simulink model "VB_RIFKF_GNSS_INS25"  (R2023a)
settings: Solver=FixedStepAuto  StartTime=0  StopTime=500  FixedStep=0.01  RelTol=1e-3
InitFcn:
  | resilient_initNavigation1216;
  | init_param;
undefined symbols (not defined in the file or in its folder): dt, g0, gam0_rad, ISUS_flag, magnitude, p, P0, P0_RIEKF, param, pd0, pe0, phi0_rad, pn0, psi, psi0_rad, state_dim, vd0, ve0, vn0
libraries: simulink_extras x68, dspstat3 x54, sharedtransform x47, simulink x43, matrix_library x9, sharedTrackingLibrary x5, dspfactors x4, aerolibconvert2 x3, aerolibtransform2 x3
(part 16 of 22)

== system VB_RIFKF_GNSS_INS25/ISUS_RIEKF3/INS propogation3/vel//pos update/Kinematic Equation ==
  Cbn : Inport
  Ab : Inport  Port=2
  Add : Sum  Inputs=+-
  Add1 : Sum  Inputs=+-
  Constant : Constant  Value=[0 0 -g0]  OutDataTypeStr=single
  Constant1 : Constant  Value=[0 0 -g0]  OutDataTypeStr=single
  Product : Product  Multiplication=Matrix(*)  RndMeth=Zero
  Product1 : Product  Multiplication=Matrix(*)  RndMeth=Zero
  Scope : Scope
  Scope1 : Scope  NumInputPorts=2
  Transpose : Math  Operator=transpose
  An : Outport
  ab_nog : Outport  Port=2
  wires:
  Cbn/1 -> Transpose/1, Product/1
  Add/1 -> An/1, Scope1/2
  Ab/1 -> Product/2, Add1/1, Scope1/1
  Product/1 -> Scope/1, Add/1
  Constant/1 -> Add/2
  Transpose/1 -> Product1/1  "Cnb"
  Constant1/1 -> Product1/2  "gn"
  Product1/1 -> Add1/2  "gb"
  Add1/1 -> ab_nog/1  "ab_nog"

== system VB_RIFKF_GNSS_INS25/ISUS_RIEKF3/INS propogation3/vel//pos update/pos update ==
  dtheta : Inport
  vel_k : Inport  Port=2
  dp : Inport  Port=3
  QGC_init : Inport  Port=4
  p0 : Inport  Port=5
  Add1 : Sum
  Delay1 : Delay  DelayLength=1  InitialConditionSource=Input port  ExternalReset=Rising
      settings: InputPortMap=u0,r5,p4
  Gain1 : Gain  Gain=dt
  MATLAB Function : MATLAB Function  TreatAsAtomicUnit=on
  Reshape1 : Reshape  OutputDimensionality=Column vector (2-D)
  p_k : Outport
  wires:
  p0/1 -> Reshape1/1
  QGC_init/1 -> Delay1/2
  Reshape1/1 -> Delay1/3
  Delay1/1 -> Add1/2
  Gain1/1 -> Add1/1
  vel_k/1 -> Gain1/1
  dtheta/1 -> MATLAB Function/1(dtheta)
  dp/1 -> MATLAB Function/2(KFState_dp)
  Add1/1 -> MATLAB Function/3(pos)
  MATLAB Function/1(pos_correct) -> Delay1/1, p_k/1

== system VB_RIFKF_GNSS_INS25/ISUS_RIEKF3/INS propogation3/vel//pos update/vel update ==
  dtheta : Inport
  QGC_init : Inport  Port=2
  An : Inport  Port=3
  KFState_dv : Inport  Port=4
  v0 : Inport  Port=5
  Add : Sum
  Delay : Delay  DelayLength=1  InitialConditionSource=Input port  ExternalReset=Rising
      settings: InputPortMap=u0,r5,p4
  Gain : Gain  Gain=dt
  MATLAB Function : MATLAB Function  TreatAsAtomicUnit=on
  Reshape : Reshape  OutputDimensionality=Column vector (2-D)
  vel_k : Outport
  wires:
  QGC_init/1 -> Delay/2
  Reshape/1 -> Delay/3
  An/1 -> Gain/1
  v0/1 -> Reshape/1
  Gain/1 -> Add/1
  Delay/1 -> Add/2
  KFState_dv/1 -> MATLAB Function/2(KFState_dv)
  dtheta/1 -> MATLAB Function/1(dtheta)
  Add/1 -> MATLAB Function/3(vel)
  MATLAB Function/1(vel_correct) -> Delay/1, vel_k/1

== system VB_RIFKF_GNSS_INS25/No.1_Sensor_Data_Process/IMU_Data_Process/Bias Eliminate/Subsystem ==
  data : Inport
  Buffer : Buffer  N=50  V=49  OutputFrames=off
  Buffer1 : Buffer  N=50  V=49  OutputFrames=off
  Buffer2 : Buffer  N=50  V=49  OutputFrames=off
  Demux : Demux  Outputs=3
  Mean4 : dspstat3/Mean  run=off  reset_popup=None  directionMode=Entire input  dimension=3  roiEnable=off  roiType=Rectangles  roiPortion=Entire ROI  roiOutput=Individual statistics for each ROI  roiFlag=off  roundingMode=Floor  overflowMode=off  outputDataTypeStr=Inherit: Same as accumulator  outputMin=[]  outputMax=[]  outputLastDataTypeStr=Inherit: Same as accumulator
  Mean5 : dspstat3/Mean  run=off  reset_popup=None  directionMode=Entire input  dimension=3  roiEnable=off  roiType=Rectangles  roiPortion=Entire ROI  roiOutput=Individual statistics for each ROI  roiFlag=off  roundingMode=Floor  overflowMode=off  outputDataTypeStr=Inherit: Same as accumulator  outputMin=[]  outputMax=[]  outputLastDataTypeStr=Inherit: Same as accumulator
  Mean6 : dspstat3/Mean  run=off  reset_popup=None  directionMode=Entire input  dimension=3  roiEnable=off  roiType=Rectangles  roiPortion=Entire ROI  roiOutput=Individual statistics for each ROI  roiFlag=off  roundingMode=Floor  overflowMode=off  outputDataTypeStr=Inherit: Same as accumulator  outputMin=[]  outputMax=[]  outputLastDataTypeStr=Inherit: Same as accumulator
  Scope : Scope  NumInputPorts=2
  Vector Concatenate : Concatenate  NumInputs=3
  mean_data : Outport
  wires:
  data/1 -> Demux/1, Scope/1
  Vector Concatenate/1 -> mean_data/1, Scope/2
  Mean4/1 -> Vector Concatenate/1
  Demux/3 -> Buffer2/1
  Buffer1/1 -> Mean5/1  "fby_buff"
  Demux/1 -> Buffer/1
  Buffer2/1 -> Mean6/1  "fbz_buff"
  Mean5/1 -> Vector Concatenate/2
  Buffer/1 -> Mean4/1  "fbx_buff"
  Demux/2 -> Buffer1/1
  Mean6/1 -> Vector Concatenate/3

== system VB_RIFKF_GNSS_INS25/No.1_Sensor_Data_Process1/IMU_Data_Process/Bias Eliminate/Subsystem ==
  data : Inport
  Buffer : Buffer  N=50  V=49  OutputFrames=off
  Buffer1 : Buffer  N=50  V=49  OutputFrames=off
  Buffer2 : Buffer  N=50  V=49  OutputFrames=off
  Demux : Demux  Outputs=3
  Mean4 : dspstat3/Mean  run=off  reset_popup=None  directionMode=Entire input  dimension=3  roiEnable=off  roiType=Rectangles  roiPortion=Entire ROI  roiOutput=Individual statistics for each ROI  roiFlag=off  roundingMode=Floor  overflowMode=off  outputDataTypeStr=Inherit: Same as accumulator  outputMin=[]  outputMax=[]  outputLastDataTypeStr=Inherit: Same as accumulator
  Mean5 : dspstat3/Mean  run=off  reset_popup=None  directionMode=Entire input  dimension=3  roiEnable=off  roiType=Rectangles  roiPortion=Entire ROI  roiOutput=Individual statistics for each ROI  roiFlag=off  roundingMode=Floor  overflowMode=off  outputDataTypeStr=Inherit: Same as accumulator  outputMin=[]  outputMax=[]  outputLastDataTypeStr=Inherit: Same as accumulator
  Mean6 : dspstat3/Mean  run=off  reset_popup=None  directionMode=Entire input  dimension=3  roiEnable=off  roiType=Rectangles  roiPortion=Entire ROI  roiOutput=Individual statistics for each ROI  roiFlag=off  roundingMode=Floor  overflowMode=off  outputDataTypeStr=Inherit: Same as accumulator  outputMin=[]  outputMax=[]  outputLastDataTypeStr=Inherit: Same as accumulator
  Scope : Scope  NumInputPorts=2
  Vector Concatenate : Concatenate  NumInputs=3
  mean_data : Outport
  wires:
  Mean6/1 -> Vector Concatenate/3
  Demux/2 -> Buffer1/1
  Buffer/1 -> Mean4/1  "fbx_buff"
  Mean5/1 -> Vector Concatenate/2
  Buffer2/1 -> Mean6/1  "fbz_buff"
  Demux/1 -> Buffer/1
  Buffer1/1 -> Mean5/1  "fby_buff"
  Demux/3 -> Buffer2/1
  Mean4/1 -> Vector Concatenate/1
  Vector Concatenate/1 -> Scope/2, mean_data/1
  data/1 -> Scope/1, Demux/1

== system VB_RIFKF_GNSS_INS25/No.1_Sensor_Data_Process2/IMU_Data_Process/Bias Eliminate/Subsystem ==
  data : Inport
  Buffer : Buffer  N=50  V=49  OutputFrames=off
  Buffer1 : Buffer  N=50  V=49  OutputFrames=off
  Buffer2 : Buffer  N=50  V=49  OutputFrames=off
  Demux : Demux  Outputs=3
  Mean4 : dspstat3/Mean  run=off  reset_popup=None  directionMode=Entire input  dimension=3  roiEnable=off  roiType=Rectangles  roiPortion=Entire ROI  roiOutput=Individual statistics for each ROI  roiFlag=off  roundingMode=Floor  overflowMode=off  outputDataTypeStr=Inherit: Same as accumulator  outputMin=[]  outputMax=[]  outputLastDataTypeStr=Inherit: Same as accumulator
  Mean5 : dspstat3/Mean  run=off  reset_popup=None  directionMode=Entire input  dimension=3  roiEnable=off  roiType=Rectangles  roiPortion=Entire ROI  roiOutput=Individual statistics for each ROI  roiFlag=off  roundingMode=Floor  overflowMode=off  outputDataTypeStr=Inherit: Same as accumulator  outputMin=[]  outputMax=[]  outputLastDataTypeStr=Inherit: Same as accumulator
  Mean6 : dspstat3/Mean  run=off  reset_popup=None  directionMode=Entire input  dimension=3  roiEnable=off  roiType=Rectangles  roiPortion=Entire ROI  roiOutput=Individual statistics for each ROI  roiFlag=off  roundingMode=Floor  overflowMode=off  outputDataTypeStr=Inherit: Same as accumulator  outputMin=[]  outputMax=[]  outputLastDataTypeStr=Inherit: Same as accumulator
  Scope : Scope  NumInputPorts=2
  Vector Concatenate : Concatenate  NumInputs=3
  mean_data : Outport
  wires:
  data/1 -> Demux/1, Scope/1
  Vector Concatenate/1 -> mean_data/1, Scope/2
  Mean4/1 -> Vector Concatenate/1
  Demux/3 -> Buffer2/1
  Buffer1/1 -> Mean5/1  "fby_buff"
  Demux/1 -> Buffer/1
  Buffer2/1 -> Mean6/1  "fbz_buff"
  Mean5/1 -> Vector Concatenate/2
  Buffer/1 -> Mean4/1  "fbx_buff"
  Demux/2 -> Buffer1/1
  Mean6/1 -> Vector Concatenate/3

== system VB_RIFKF_GNSS_INS25/ER EKF/Error State Kalman Filter/Extended Kalman Filter1/Correct1/Sk_m_innovation ==
  Pk/k_1 : Inport
  yMeas : Inport  Port=2
  X : Inport  Port=3
  R : Inport  Port=4
  Abs : Abs  Commented=on  SaturateOnIntegerOverflow=off
  Abs1 : Abs  SaturateOnIntegerOverflow=off
  Add : Sum
  Add1 : Sum  Inputs=+-
  Add2 : Sum
  Constant : Constant  Commented=on  Value=8
  Constant1 : Constant  Commented=on  Value=8
  Constant2 : Constant  Commented=on  Value=12
  Constant3 : Constant  Value=eps
  Constant4 : Constant  Commented=on  Value=15
  Constant5 : Constant  Commented=on  Value=8
  Constant6 : Constant  Value=[eye(6),zeros(6,9)]  OutDataTypeStr=single
  Constant7 : Constant  Commented=on  Value=15
  Constant8 : Constant  Commented=on  Value=12
  Constant9 : Constant  Commented=on  Value=25
  Divide : Product  Inputs=*/
  Extract Diagonal1 : matrix_library/Extract Diagonal
  MATLAB Function : MATLAB Function  Commented=on  TreatAsAtomicUnit=on
  Product : Product  Inputs=3  Multiplication=Matrix(*)
  Product1 : Product  Multiplication=Matrix(*)
  Product2 : Product  Commented=on
  Scope : Scope
  Sqrt1 : Sqrt
  Transpose : Math  Operator=transpose
  yMeas1 : InportShadow  Port=2
  measurement innovation : Outport
  wires:
  Product/1 -> Add/1
  Transpose/1 -> Product/3
  R/1 -> Add/2
  Pk/k_1/1 -> Product/2
  yMeas/1 -> Add1/1
  Constant6/1 -> Product1/1, Product/1, Transpose/1
  X/1 -> Product1/2
  Product1/1 -> Add1/2
  Add/1 -> Extract Diagonal1/1  "S"
  Divide/1 -> measurement innovation/1, Abs/1, Scope/1
  MATLAB Function/1(w) -> Product2/1
  Extract Diagonal1/1 -> Abs1/1
  Add1/1 -> Divide/1
  Sqrt1/1 -> Add2/1
  Abs/1 -> MATLAB Function/1(err)
  Abs1/1 -> Sqrt1/1
  Add2/1 -> Divide/2
  Constant3/1 -> Add2/2
  yMeas1/1 -> Product2/2
  Constant1/1 -> MATLAB Function/2(k0)
  Constant4/1 -> MATLAB Function/3(k1)
  Constant/1 -> MATLAB Function/4(zk0)
  Constant2/1 -> MATLAB Function/5(zk1)

== system VB_RIFKF_GNSS_INS25/ER EKF/Error State Kalman Filter/Extended Kalman Filter1/Predict/If Action Subsystem ==
  Action Port : ActionPort
  Constant : Constant  Value=0
  Data Store Read : DataStoreRead  DataStoreName=x  IndexOptions=Index vector (dialog)  Indices=1  OutputSizes=1
  Data Store Write : DataStoreWrite  DataStoreName=x  IndexOptions=Index vector (dialog)  Indices=1  OutputSizes=1
  Data Store Write1 : DataStoreWrite  DataStoreName=feedback_flag_18dim  IndexOptions=Index vector (dialog)  Indices=1  OutputSizes=1
  Mux : Mux  Inputs=2
  Selector : Selector  InputPortWidth=18  IndexOptions=Index vector (dialog)  Indices=[16 17 18]  OutputSizes=1
  Zero : Constant  Value=zeros(15,1)  OutDataTypeStr=Inherit: Inherit via back propagation
  wires:
  Constant/1 -> Data Store Write1/1
  Data Store Read/1 -> Selector/1
  Zero/1 -> Mux/1
  Selector/1 -> Mux/2
  Mux/1 -> Data Store Write/1

== system VB_RIFKF_GNSS_INS25/ER EKF/Error State Kalman Filter/Extended Kalman Filter2/Correct1/Sk_m_innovation ==
  Pk/k_1 : Inport
  yMeas : Inport  Port=2
  X : Inport  Port=3
  R : Inport  Port=4
  Abs : Abs  Commented=on  SaturateOnIntegerOverflow=off
  Abs1 : Abs  SaturateOnIntegerOverflow=off
  Add : Sum
  Add1 : Sum  Inputs=+-
  Add2 : Sum
  Constant : Constant  Commented=on  Value=8
  Constant1 : Constant  Commented=on  Value=8
  Constant2 : Constant  Commented=on  Value=12
  Constant3 : Constant  Value=eps
  Constant4 : Constant  Commented=on  Value=15
  Constant5 : Constant  Commented=on  Value=8
  Constant6 : Constant  Value=[eye(6),zeros(6,9)]  OutDataTypeStr=single
  Constant7 : Constant  Commented=on  Value=15
  Constant8 : Constant  Commented=on  Value=12
  Constant9 : Constant  Commented=on  Value=25
  Divide : Product  Inputs=*/
  Extract Diagonal1 : matrix_library/Extract Diagonal
  MATLAB Function : MATLAB Function  Commented=on  TreatAsAtomicUnit=on
  Product : Product  Inputs=3  Multiplication=Matrix(*)
  Product1 : Product  Multiplication=Matrix(*)
  Product2 : Product  Commented=on
  Scope : Scope
  Sqrt1 : Sqrt
  Transpose : Math  Operator=transpose
  yMeas1 : InportShadow  Port=2
  measurement innovation : Outport
  wires:
  Product/1 -> Add/1
  Transpose/1 -> Product/3
  R/1 -> Add/2
  Pk/k_1/1 -> Product/2
  yMeas/1 -> Add1/1
  Constant6/1 -> Product1/1, Product/1, Transpose/1
  X/1 -> Product1/2
  Product1/1 -> Add1/2
  Add/1 -> Extract Diagonal1/1  "S"
  Divide/1 -> measurement innovation/1, Abs/1, Scope/1
  MATLAB Function/1(w) -> Product2/1
  Extract Diagonal1/1 -> Abs1/1
  Add1/1 -> Divide/1
  Sqrt1/1 -> Add2/1
  Abs/1 -> MATLAB Function/1(err)
  Abs1/1 -> Sqrt1/1
  Add2/1 -> Divide/2
  Constant3/1 -> Add2/2
  yMeas1/1 -> Product2/2
  Constant1/1 -> MATLAB Function/2(k0)
  Constant4/1 -> MATLAB Function/3(k1)
  Constant/1 -> MATLAB Function/4(zk0)
  Constant2/1 -> MATLAB Function/5(zk1)

== system VB_RIFKF_GNSS_INS25/ER EKF/Error State Kalman Filter/Extended Kalman Filter2/Predict/If Action Subsystem ==
  Action Port : ActionPort
  Constant : Constant  Value=0
  Data Store Read : DataStoreRead  DataStoreName=x  IndexOptions=Index vector (dialog)  Indices=1  OutputSizes=1
  Data Store Write : DataStoreWrite  DataStoreName=x  IndexOptions=Index vector (dialog)  Indices=1  OutputSizes=1
  Data Store Write1 : DataStoreWrite  DataStoreName=feedback_flag_18dim  IndexOptions=Index vector (dialog)  Indices=1  OutputSizes=1
  Mux : Mux  Inputs=2
  Selector : Selector  InputPortWidth=18  IndexOptions=Index vector (dialog)  Indices=[16 17 18]  OutputSizes=1
  Zero : Constant  Value=zeros(15,1)  OutDataTypeStr=Inherit: Inherit via back propagation
  wires:
  Constant/1 -> Data Store Write1/1
  Data Store Read/1 -> Selector/1
  Zero/1 -> Mux/1
  Selector/1 -> Mux/2
  Mux/1 -> Data Store Write/1

== system VB_RIFKF_GNSS_INS25/ER EKF/INS propogation/Init_PVQ/Horizontal_attitude/Deal with zero ==
  In1 : Inport
  Add5 : Sum
  Constant1 : Constant  Value=1e-6  OutDataTypeStr=single
  Out1 : Outport
  wires:
  Constant1/1 -> Add5/2
  In1/1 -> Add5/1
  Add5/1 -> Out1/1

== system VB_RIFKF_GNSS_INS25/ER EKF/INS propogation/Init_PVQ/Horizontal_attitude2/Deal with zero ==
  In1 : Inport
  Add5 : Sum
  Constant1 : Constant  Value=1e-6  OutDataTypeStr=single
  Out1 : Outport
  wires:
  Constant1/1 -> Add5/2
  In1/1 -> Add5/1
  Add5/1 -> Out1/1

== system VB_RIFKF_GNSS_INS25/ER EKF/INS propogation/gyro bias compensation/error compensation/If Action Subsystem1 ==
  Action Port : ActionPort  ActionPortLabel=if(u1 == 1)
  Constant : Constant
  Data Store Write : DataStoreWrite  DataStoreName=feedback_flag_18dim  IndexOptions=Index vector (dialog)  Indices=1  OutputSizes=1
  wires:
  Constant/1 -> Data Store Write/1

== system VB_RIFKF_GNSS_INS25/ISUS_RIEKF1/Error State Kalman Filter M1/Extended Kalman Filter M1/Predict/If Action Subsystem ==
  Action Port : ActionPort
  Constant : Constant  Value=0
  Data Store Read : DataStoreRead  DataStoreName=x  IndexOptions=Index vector (dialog)  Indices=1  OutputSizes=1
  Data Store Write : DataStoreWrite  DataStoreName=x  IndexOptions=Index vector (dialog)  Indices=1  OutputSizes=1
  Data Store Write1 : DataStoreWrite  DataStoreName=feedback_flag_18dim  IndexOptions=Index vector (dialog)  Indices=1  OutputSizes=1
  Mux : Mux  Inputs=2
  Selector : Selector  InputPortWidth=18  IndexOptions=Index vector (dialog)  Indices=[16 17 18]  OutputSizes=1
  Zero : Constant  Value=zeros(15,1)  OutDataTypeStr=Inherit: Inherit via back propagation
  wires:
  Constant/1 -> Data Store Write1/1
  Data Store Read/1 -> Selector/1
  Zero/1 -> Mux/1
  Selector/1 -> Mux/2
  Mux/1 -> Data Store Write/1

== system VB_RIFKF_GNSS_INS25/ISUS_RIEKF1/Error State Kalman Filter M1/Extended Kalman Filter M2/Predict/If Action Subsystem ==
  Action Port : ActionPort
  Constant : Constant  Value=0
  Data Store Read : DataStoreRead  DataStoreName=x  IndexOptions=Index vector (dialog)  Indices=1  OutputSizes=1
  Data Store Write : DataStoreWrite  DataStoreName=x  IndexOptions=Index vector (dialog)  Indices=1  OutputSizes=1
  Data Store Write1 : DataStoreWrite  DataStoreName=feedback_flag_18dim  IndexOptions=Index vector (dialog)  Indices=1  OutputSizes=1
  Mux : Mux  Inputs=2
  Selector : Selector  InputPortWidth=18  IndexOptions=Index vector (dialog)  Indices=[16 17 18]  OutputSizes=1
  Zero : Constant  Value=zeros(15,1)  OutDataTypeStr=Inherit: Inherit via back propagation
  wires:
  Mux/1 -> Data Store Write/1
  Selector/1 -> Mux/2
  Zero/1 -> Mux/1
  Data Store Read/1 -> Selector/1
  Constant/1 -> Data Store Write1/1

== system VB_RIFKF_GNSS_INS25/ISUS_RIEKF1/Error State Kalman Filter M1/bak/Simulink Function - State Transition Jacobian/Cal Phi1 ==
  Rbn : Inport
  vn : Inport  Port=2
  pn : Inport  Port=3
  Constant : Constant  Value=dt
  MATLAB Function1 : MATLAB Function  TreatAsAtomicUnit=on
  Reshape : Reshape  OutputDimensionality=Column vector (2-D)
  Reshape1 : Reshape  OutputDimensionality=Column vector (2-D)
  Phi : Outport
  wires:
  Reshape1/1 -> MATLAB Function1/2(pn)
  Reshape/1 -> MATLAB Function1/1(vn)
  pn/1 -> Reshape1/1
  vn/1 -> Reshape/1
  Rbn/1 -> MATLAB Function1/3(Rbn)
  MATLAB Function1/1(Phi) -> Phi/1
  Constant/1 -> MATLAB Function1/4(dt)

== system VB_RIFKF_GNSS_INS25/ISUS_RIEKF1/INS propogation/Init_PVQ/Horizontal_attitude/Deal with zero ==
  In1 : Inport
  Add5 : Sum
  Constant1 : Constant  Value=1e-6  OutDataTypeStr=single
  Out1 : Outport
  wires:
  Constant1/1 -> Add5/2
  In1/1 -> Add5/1
  Add5/1 -> Out1/1

== system VB_RIFKF_GNSS_INS25/ISUS_RIEKF1/INS propogation/gyro bias compensation/error compensation/If Action Subsystem1 ==
  Action Port : ActionPort  ActionPortLabel=if(u1 == 1)
  Constant : Constant
  Data Store Write : DataStoreWrite  DataStoreName=feedback_flag_18dim_RIEKF  IndexOptions=Index vector (dialog)  Indices=1  OutputSizes=1
  wires:
  Constant/1 -> Data Store Write/1

== system VB_RIFKF_GNSS_INS25/ISUS_RIEKF2/Error State Kalman Filter M1/Extended Kalman Filter M1/Predict/If Action Subsystem ==
  Action Port : ActionPort
  Constant : Constant  Value=0
  Data Store Read : DataStoreRead  DataStoreName=x  IndexOptions=Index vector (dialog)  Indices=1  OutputSizes=1
  Data Store Write : DataStoreWrite  DataStoreName=x  IndexOptions=Index vector (dialog)  Indices=1  OutputSizes=1
  Data Store Write1 : DataStoreWrite  DataStoreName=feedback_flag_18dim  IndexOptions=Index vector (dialog)  Indices=1  OutputSizes=1
  Mux : Mux  Inputs=2
  Selector : Selector  InputPortWidth=18  IndexOptions=Index vector (dialog)  Indices=[16 17 18]  OutputSizes=1
  Zero : Constant  Value=zeros(15,1)  OutDataTypeStr=Inherit: Inherit via back propagation
  wires:
  Mux/1 -> Data Store Write/1
  Selector/1 -> Mux/2
  Zero/1 -> Mux/1
  Data Store Read/1 -> Selector/1
  Constant/1 -> Data Store Write1/1

== system VB_RIFKF_GNSS_INS25/ISUS_RIEKF2/Error State Kalman Filter M1/bak/Simulink Function - State Transition Jacobian/Cal Phi1 ==
  Rbn : Inport
  vn : Inport  Port=2
  pn : Inport  Port=3
  Constant : Constant  Value=dt
  MATLAB Function1 : MATLAB Function  TreatAsAtomicUnit=on
  Reshape : Reshape  OutputDimensionality=Column vector (2-D)
  Reshape1 : Reshape  OutputDimensionality=Column vector (2-D)
  Phi : Outport
  wires:
  Constant/1 -> MATLAB Function1/4(dt)
  MATLAB Function1/1(Phi) -> Phi/1
  Rbn/1 -> MATLAB Function1/3(Rbn)
  vn/1 -> Reshape/1
  pn/1 -> Reshape1/1
  Reshape/1 -> MATLAB Function1/1(vn)
  Reshape1/1 -> MATLAB Function1/2(pn)

== system VB_RIFKF_GNSS_INS25/ISUS_RIEKF2/INS propogation/Init_PVQ/Horizontal_attitude/Deal with zero ==
  In1 : Inport
  Add5 : Sum
  Constant1 : Constant  Value=1e-6  OutDataTypeStr=single
  Out1 : Outport
  wires:
  Add5/1 -> Out1/1
  In1/1 -> Add5/1
  Constant1/1 -> Add5/2

== system VB_RIFKF_GNSS_INS25/ISUS_RIEKF2/INS propogation/gyro bias compensation/error compensation/If Action Subsystem1 ==
  Action Port : ActionPort  ActionPortLabel=if(u1 == 1)
  Constant : Constant
  Data Store Write : DataStoreWrite  DataStoreName=feedback_flag_18dim_RIEKF  IndexOptions=Index vector (dialog)  Indices=1  OutputSizes=1
  wires:
  Constant/1 -> Data Store Write/1

== system VB_RIFKF_GNSS_INS25/ISUS_RIEKF3/Error State Kalman Filter M1/Extended Kalman Filter M1/Correct M1/Subsystem2 ==
  Pk_1_ISIU : Inport
  Pk_2 : Inport  Port=2
  Constant : Constant  Value=ISUS_flag
  Data Type Conversion : DataTypeConversion  OutDataTypeStr=single  SaturateOnIntegerOverflow=off  RndMeth=Floor
  MATLAB Function1 : MATLAB Function  TreatAsAtomicUnit=on
  Scope : Scope
  y1 : Outport
  wires:
  MATLAB Function1/1(y) -> y1/1
  Pk_1_ISIU/1 -> Data Type Conversion/1
  Pk_2/1 -> MATLAB Function1/2(X)
  Constant/1 -> Scope/1, MATLAB Function1/3(ISUS_flag)
  Data Type Conversion/1 -> MATLAB Function1/1(u)

== system VB_RIFKF_GNSS_INS25/ISUS_RIEKF3/Error State Kalman Filter M1/Extended Kalman Filter M1/Correct M1/innovation calculation ==
  Pk/k_1 : Inport
  yMeas : Inport  Port=2
  X : Inport  Port=3
  R : Inport  Port=4
  H : Inport  Port=5
  Add : Sum
  Add1 : Sum  Inputs=+-
  MATLAB Function : MATLAB Function  TreatAsAtomicUnit=on
  Product : Product  Inputs=3  Multiplication=Matrix(*)
  Product1 : Product  Multiplication=Matrix(*)
  Scope1 : Scope
  Scope2 : Scope
  Transpose : Math  Operator=transpose
  Sk : Outport
  m_innov : Outport  Port=2
  wires:
  MATLAB Function/1(y) -> Product/2
  Product/1 -> Add/1
  Transpose/1 -> Product/3
  R/1 -> Add/2
  Pk/k_1/1 -> MATLAB Function/1(u)
  yMeas/1 -> Add1/1
  H/1 -> Product1/1, Product/1, Transpose/1
  X/1 -> Product1/2, Scope2/1
  Product1/1 -> Add1/2
  Add/1 -> Sk/1  "S"
  Add1/1 -> m_innov/1, Scope1/1

== system VB_RIFKF_GNSS_INS25/ISUS_RIEKF3/Error State Kalman Filter M1/Extended Kalman Filter M1/Correct M1/innovation calculation1 ==
  note: 20250411
      | 计算故障检测函数值Gamma
  Pk/k_1 : Inport
  yMeas : Inport  Port=2
  X : Inport  Port=3
  H : Inport  Port=4
  Rk1 : Inport  Port=5
  Add : Sum
  Add1 : Sum  Inputs=+-
  Cast To Double : DataTypeConversion  OutDataTypeStr=single  SaturateOnIntegerOverflow=off  RndMeth=Floor
  Display : Display
  Display3 : Display
  Display6 : Display
  MATLAB Function : MATLAB Function  TreatAsAtomicUnit=on
  MATLAB Function1 : MATLAB Function  TreatAsAtomicUnit=on
  MATLAB Function3 : MATLAB Function  TreatAsAtomicUnit=on
  Product : Product  Inputs=3  Multiplication=Matrix(*)
  Product1 : Product  Multiplication=Matrix(*)
  Product2 : Product  Multiplication=Matrix(*)
  Scope{,1..3} (4 alike) : Scope
  Transpose : Math  Operator=transpose
  Transpose1 : Math  Operator=transpose
  Sk : Outport
  m_innov : Outport  Port=2
  beta : Outport  Port=3
  wires:
  MATLAB Function/1(y) -> Product/2
  Product/1 -> Add/1
  Transpose/1 -> Product/3
  Pk/k_1/1 -> MATLAB Function/1(u)
  yMeas/1 -> Add1/1
  H/1 -> Product1/1, Product/1, Transpose/1
  X/1 -> Product1/2, Scope2/1
  Product1/1 -> Add1/2
  Add/1 -> MATLAB Function3/2(S), MATLAB Function1/2(S), Sk/1  "S"
  Add1/1 -> MATLAB Function3/1(r), Product2/2, Transpose1/1, Display6/1, m_innov/1, Scope1/1
  Transpose1/1 -> Product2/1
  Product2/1 -> MATLAB Function1/1(r), Display3/1
  MATLAB Function1/1(beta) -> Display/1, Cast To Double/1
  Cast To Double/1 -> beta/1
  Rk1/1 -> Add/2
  MATLAB Function1/2(deltaV) -> Scope/1
  MATLAB Function3/1(Gamma) -> Scope3/1

== system VB_RIFKF_GNSS_INS25/ISUS_RIEKF3/Error State Kalman Filter M1/Extended Kalman Filter M1/Predict/If Action Subsystem ==
  Action Port : ActionPort
  Constant : Constant  Value=0
  Data Store Read : DataStoreRead  DataStoreName=x  IndexOptions=Index vector (dialog)  Indices=1  OutputSizes=1
  Data Store Write : DataStoreWrite  DataStoreName=x  IndexOptions=Index vector (dialog)  Indices=1  OutputSizes=1
  Data Store Write1 : DataStoreWrite  DataStoreName=feedback_flag_18dim  IndexOptions=Index vector (dialog)  Indices=1  OutputSizes=1
  Mux : Mux  Inputs=2
  Selector : Selector  InputPortWidth=18  IndexOptions=Index vector (dialog)  Indices=[16 17 18]  OutputSizes=1
  Zero : Constant  Value=zeros(15,1)  OutDataTypeStr=Inherit: Inherit via back propagation
  wires:
  Constant/1 -> Data Store Write1/1
  Data Store Read/1 -> Selector/1
  Zero/1 -> Mux/1
  Selector/1 -> Mux/2
  Mux/1 -> Data Store Write/1

== system VB_RIFKF_GNSS_INS25/ISUS_RIEKF3/Error State Kalman Filter M1/VB-Extended Kalman Filter M2/Correct M1/Subsystem2 ==
  Pk_1_ISIU : Inport
  Pk_2 : Inport  Port=2
  Constant : Constant  Value=ISUS_flag
  Data Type Conversion : DataTypeConversion  OutDataTypeStr=single  SaturateOnIntegerOverflow=off  RndMeth=Floor
  MATLAB Function1 : MATLAB Function  TreatAsAtomicUnit=on
  Scope : Scope
  y1 : Outport
  wires:
  Data Type Conversion/1 -> MATLAB Function1/1(u)
  Constant/1 -> MATLAB Function1/3(ISUS_flag), Scope/1
  Pk_2/1 -> MATLAB Function1/2(X)
  Pk_1_ISIU/1 -> Data Type Conversion/1
  MATLAB Function1/1(y) -> y1/1

== system VB_RIFKF_GNSS_INS25/ISUS_RIEKF3/Error State Kalman Filter M1/VB-Extended Kalman Filter M2/Correct M1/innovation calculation ==
  Pk/k_1 : Inport
  yMeas : Inport  Port=2
  X : Inport  Port=3
  R : Inport  Port=4
  H : Inport  Port=5
  Add : Sum
  Add1 : Sum  Inputs=+-
  MATLAB Function : MATLAB Function  TreatAsAtomicUnit=on
  Product : Product  Inputs=3  Multiplication=Matrix(*)
  Product1 : Product  Multiplication=Matrix(*)
  Scope1 : Scope
  Scope2 : Scope
  Transpose : Math  Operator=transpose
  Sk : Outport
  m_innov : Outport  Port=2
  wires:
  Add1/1 -> Scope1/1, m_innov/1
  Add/1 -> Sk/1  "S"
  Product1/1 -> Add1/2
  X/1 -> Scope2/1, Product1/2
  H/1 -> Transpose/1, Product/1, Product1/1
  yMeas/1 -> Add1/1
  Pk/k_1/1 -> MATLAB Function/1(u)
  R/1 -> Add/2
  Transpose/1 -> Product/3
  Product/1 -> Add/1
  MATLAB Function/1(y) -> Product/2

== system VB_RIFKF_GNSS_INS25/ISUS_RIEKF3/Error State Kalman Filter M1/VB-Extended Kalman Filter M2/Predict/If Action Subsystem ==
  Action Port : ActionPort
  Constant : Constant  Value=0
  Data Store Read : DataStoreRead  DataStoreName=x  IndexOptions=Index vector (dialog)  Indices=1  OutputSizes=1
  Data Store Write : DataStoreWrite  DataStoreName=x  IndexOptions=Index vector (dialog)  Indices=1  OutputSizes=1
  Data Store Write1 : DataStoreWrite  DataStoreName=feedback_flag_18dim  IndexOptions=Index vector (dialog)  Indices=1  OutputSizes=1
  Mux : Mux  Inputs=2
  Selector : Selector  InputPortWidth=18  IndexOptions=Index vector (dialog)  Indices=[16 17 18]  OutputSizes=1
  Zero : Constant  Value=zeros(15,1)  OutDataTypeStr=Inherit: Inherit via back propagation
  wires:
  Mux/1 -> Data Store Write/1
  Selector/1 -> Mux/2
  Zero/1 -> Mux/1
  Data Store Read/1 -> Selector/1
  Constant/1 -> Data Store Write1/1

== system VB_RIFKF_GNSS_INS25/ISUS_RIEKF3/Error State Kalman Filter M1/bak/Simulink Function - State Transition Jacobian/Cal Phi1 ==
  Rbn : Inport
  vn : Inport  Port=2
  pn : Inport  Port=3
  Constant : Constant  Value=dt
  MATLAB Function1 : MATLAB Function  TreatAsAtomicUnit=on
  Reshape : Reshape  OutputDimensionality=Column vector (2-D)
  Reshape1 : Reshape  OutputDimensionality=Column vector (2-D)
  Phi : Outport
  wires:
  Reshape1/1 -> MATLAB Function1/2(pn)
  Reshape/1 -> MATLAB Function1/1(vn)
  pn/1 -> Reshape1/1
  vn/1 -> Reshape/1
  Rbn/1 -> MATLAB Function1/3(Rbn)
  MATLAB Function1/1(Phi) -> Phi/1
  Constant/1 -> MATLAB Function1/4(dt)

== system VB_RIFKF_GNSS_INS25/ISUS_RIEKF3/Error State Kalman Filter M2/Extended Kalman Filter M1/Correct M1/Subsystem2 ==
  Pk_1_ISIU : Inport
  Pk_2 : Inport  Port=2
  Constant : Constant  Value=ISUS_flag
  Data Type Conversion : DataTypeConversion  OutDataTypeStr=single  SaturateOnIntegerOverflow=off  RndMeth=Floor
  MATLAB Function1 : MATLAB Function  TreatAsAtomicUnit=on
  y1 : Outport
  wires:
  Data Type Conversion/1 -> MATLAB Function1/1(u)
  Constant/1 -> MATLAB Function1/3(ISUS_flag)
  Pk_2/1 -> MATLAB Function1/2(X)
  Pk_1_ISIU/1 -> Data Type Conversion/1
  MATLAB Function1/1(y) -> y1/1

== system VB_RIFKF_GNSS_INS25/ISUS_RIEKF3/Error State Kalman Filter M2/Extended Kalman Filter M1/Correct M1/innovation calculation ==
  Pk/k_1 : Inport
  yMeas : Inport  Port=2
  X : Inport  Port=3
  R : Inport  Port=4
  H : Inport  Port=5
  Add : Sum
  Add1 : Sum  Inputs=+-
  MATLAB Function : MATLAB Function  TreatAsAtomicUnit=on
  Product : Product  Inputs=3  Multiplication=Matrix(*)
  Product1 : Product  Multiplication=Matrix(*)
  Scope1 : Scope
  Scope2 : Scope
  Scope3 : Scope  NumInputPorts=2
  Selector : Selector  InputPortWidth=6  IndexOptions=Index vector (dialog)  Indices=[4]  OutputSizes=1
  Selector1 : Selector  InputPortWidth=6  IndexOptions=Index vector (dialog)  Indices=[4]  OutputSizes=1
  Transpose : Math  Operator=transpose
  Sk : Outport
  m_innov : Outport  Port=2
  wires:
  Selector1/1 -> Scope3/2
  Selector/1 -> Scope3/1
  Add1/1 -> Scope1/1, m_innov/1, Selector1/1
  Add/1 -> Sk/1  "S"
  Product1/1 -> Add1/2
  X/1 -> Scope2/1, Product1/2
  H/1 -> Transpose/1, Product/1, Product1/1
  yMeas/1 -> Add1/1, Selector/1
  Pk/k_1/1 -> MATLAB Function/1(u)
  R/1 -> Add/2
  Transpose/1 -> Product/3
  Product/1 -> Add/1
  MATLAB Function/1(y) -> Product/2

== system VB_RIFKF_GNSS_INS25/ISUS_RIEKF3/Error State Kalman Filter M2/Extended Kalman Filter M1/Predict/If Action Subsystem ==
  Action Port : ActionPort
  Constant : Constant  Value=0
  Data Store Read : DataStoreRead  DataStoreName=x  IndexOptions=Index vector (dialog)  Indices=1  OutputSizes=1
  Data Store Write : DataStoreWrite  DataStoreName=x  IndexOptions=Index vector (dialog)  Indices=1  OutputSizes=1
  Data Store Write1 : DataStoreWrite  DataStoreName=feedback_flag_18dim  IndexOptions=Index vector (dialog)  Indices=1  OutputSizes=1
  Mux : Mux  Inputs=2
  Selector : Selector  InputPortWidth=18  IndexOptions=Index vector (dialog)  Indices=[16 17 18]  OutputSizes=1
  Zero : Constant  Value=zeros(15,1)  OutDataTypeStr=Inherit: Inherit via back propagation
  wires:
  Mux/1 -> Data Store Write/1
  Selector/1 -> Mux/2
  Zero/1 -> Mux/1
  Data Store Read/1 -> Selector/1
  Constant/1 -> Data Store Write1/1

== system VB_RIFKF_GNSS_INS25/ISUS_RIEKF3/Error State Kalman Filter M2/bak/Simulink Function - State Transition Jacobian/Cal Phi1 ==
  Rbn : Inport
  vn : Inport  Port=2
  pn : Inport  Port=3
  Constant : Constant  Value=dt
  MATLAB Function1 : MATLAB Function  TreatAsAtomicUnit=on
  Reshape : Reshape  OutputDimensionality=Column vector (2-D)
  Reshape1 : Reshape  OutputDimensionality=Column vector (2-D)
  Phi : Outport
  wires:
  Constant/1 -> MATLAB Function1/4(dt)
  MATLAB Function1/1(Phi) -> Phi/1
  Rbn/1 -> MATLAB Function1/3(Rbn)
  vn/1 -> Reshape/1
  pn/1 -> Reshape1/1
  Reshape/1 -> MATLAB Function1/1(vn)
  Reshape1/1 -> MATLAB Function1/2(pn)

== system VB_RIFKF_GNSS_INS25/ISUS_RIEKF3/Error State Kalman Filter M3/Extended Kalman Filter M1/Correct M1/Subsystem2 ==
  Pk_1_ISIU : Inport
  Pk_2 : Inport  Port=2
  Constant : Constant  Value=ISUS_flag
  Data Type Conversion : DataTypeConversion  OutDataTypeStr=single  SaturateOnIntegerOverflow=off  RndMeth=Floor
  MATLAB Function1 : MATLAB Function  TreatAsAtomicUnit=on
  y1 : Outport
  wires:
  MATLAB Function1/1(y) -> y1/1
  Pk_1_ISIU/1 -> Data Type Conversion/1
  Pk_2/1 -> MATLAB Function1/2(X)
  Constant/1 -> MATLAB Function1/3(ISUS_flag)
  Data Type Conversion/1 -> MATLAB Function1/1(u)

== system VB_RIFKF_GNSS_INS25/ISUS_RIEKF3/Error State Kalman Filter M3/Extended Kalman Filter M1/Correct M1/innovation calculation ==
  Pk/k_1 : Inport
  yMeas : Inport  Port=2
  X : Inport  Port=3
  R : Inport  Port=4
  H : Inport  Port=5
  Add : Sum
  Add1 : Sum  Inputs=+-
  MATLAB Function : MATLAB Function  TreatAsAtomicUnit=on
  Product : Product  Inputs=3  Multiplication=Matrix(*)
  Product1 : Product  Multiplication=Matrix(*)
  Scope1 : Scope
  Scope2 : Scope
  Scope3 : Scope  NumInputPorts=2
  Selector : Selector  InputPortWidth=6  IndexOptions=Index vector (dialog)  Indices=[4]  OutputSizes=1
  Selector1 : Selector  InputPortWidth=6  IndexOptions=Index vector (dialog)  Indices=[4]  OutputSizes=1
  Transpose : Math  Operator=transpose
  Sk : Outport
  m_innov : Outport  Port=2
  wires:
  MATLAB Function/1(y) -> Product/2
  Product/1 -> Add/1
  Transpose/1 -> Product/3
  R/1 -> Add/2
  Pk/k_1/1 -> MATLAB Function/1(u)
  yMeas/1 -> Selector/1, Add1/1
  H/1 -> Product1/1, Product/1, Transpose/1
  X/1 -> Product1/2, Scope2/1
  Product1/1 -> Add1/2
  Add/1 -> Sk/1  "S"
  Add1/1 -> Selector1/1, m_innov/1, Scope1/1
  Selector/1 -> Scope3/1
  Selector1/1 -> Scope3/2

== system VB_RIFKF_GNSS_INS25/ISUS_RIEKF3/Error State Kalman Filter M3/Extended Kalman Filter M1/Predict/If Action Subsystem ==
  Action Port : ActionPort
  Constant : Constant  Value=0
  Data Store Read : DataStoreRead  DataStoreName=x  IndexOptions=Index vector (dialog)  Indices=1  OutputSizes=1
  Data Store Write : DataStoreWrite  DataStoreName=x  IndexOptions=Index vector (dialog)  Indices=1  OutputSizes=1
  Data Store Write1 : DataStoreWrite  DataStoreName=feedback_flag_18dim  IndexOptions=Index vector (dialog)  Indices=1  OutputSizes=1
  Mux : Mux  Inputs=2
  Selector : Selector  InputPortWidth=18  IndexOptions=Index vector (dialog)  Indices=[16 17 18]  OutputSizes=1
  Zero : Constant  Value=zeros(15,1)  OutDataTypeStr=Inherit: Inherit via back propagation
  wires:
  Constant/1 -> Data Store Write1/1
  Data Store Read/1 -> Selector/1
  Zero/1 -> Mux/1
  Selector/1 -> Mux/2
  Mux/1 -> Data Store Write/1

== system VB_RIFKF_GNSS_INS25/ISUS_RIEKF3/Error State Kalman Filter M3/bak/Simulink Function - State Transition Jacobian/Cal Phi1 ==
  Rbn : Inport
  vn : Inport  Port=2
  pn : Inport  Port=3
  Constant : Constant  Value=dt
  MATLAB Function1 : MATLAB Function  TreatAsAtomicUnit=on
  Reshape : Reshape  OutputDimensionality=Column vector (2-D)
  Reshape1 : Reshape  OutputDimensionality=Column vector (2-D)
  Phi : Outport
  wires:
  Reshape1/1 -> MATLAB Function1/2(pn)
  Reshape/1 -> MATLAB Function1/1(vn)
  pn/1 -> Reshape1/1
  vn/1 -> Reshape/1
  Rbn/1 -> MATLAB Function1/3(Rbn)
  MATLAB Function1/1(Phi) -> Phi/1
  Constant/1 -> MATLAB Function1/4(dt)

== system VB_RIFKF_GNSS_INS25/ISUS_RIEKF3/INS propogation/Init_PVQ/Horizontal_attitude/Deal with zero ==
  In1 : Inport
  Add5 : Sum
  Constant1 : Constant  Value=1e-6  OutDataTypeStr=single
  Out1 : Outport
  wires:
  Constant1/1 -> Add5/2
  In1/1 -> Add5/1
  Add5/1 -> Out1/1

== system VB_RIFKF_GNSS_INS25/ISUS_RIEKF3/INS propogation/gyro bias compensation/error compensation/If Action Subsystem1 ==
  Action Port : ActionPort  ActionPortLabel=if(u1 == 1)
  Constant : Constant
  Data Store Write : DataStoreWrite  DataStoreName=feedback_flag_18dim_RIEKF  IndexOptions=Index vector (dialog)  Indices=1  OutputSizes=1
  wires:
  Constant/1 -> Data Store Write/1

== system VB_RIFKF_GNSS_INS25/ISUS_RIEKF3/INS propogation1/Init_PVQ/Horizontal_attitude/Deal with zero ==
  In1 : Inport
  Add5 : Sum
  Constant1 : Constant  Value=1e-6  OutDataTypeStr=single
  Out1 : Outport
  wires:
  Add5/1 -> Out1/1
  In1/1 -> Add5/1
  Constant1/1 -> Add5/2

== system VB_RIFKF_GNSS_INS25/ISUS_RIEKF3/INS propogation1/gyro bias compensation/error compensation/If Action Subsystem1 ==
  Action Port : ActionPort  ActionPortLabel=if(u1 == 1)
  Constant : Constant
  Data Store Write : DataStoreWrite  DataStoreName=feedback_flag_18dim_RIEKF  IndexOptions=Index vector (dialog)  Indices=1  OutputSizes=1
  wires:
  Constant/1 -> Data Store Write/1

== system VB_RIFKF_GNSS_INS25/ISUS_RIEKF3/INS propogation2/Init_PVQ/Horizontal_attitude/Deal with zero ==
  In1 : Inport
  Add5 : Sum
  Constant1 : Constant  Value=1e-6  OutDataTypeStr=single
  Out1 : Outport
  wires:
  Constant1/1 -> Add5/2
  In1/1 -> Add5/1
  Add5/1 -> Out1/1

== system VB_RIFKF_GNSS_INS25/ISUS_RIEKF3/INS propogation2/gyro bias compensation/error compensation/If Action Subsystem1 ==
  Action Port : ActionPort  ActionPortLabel=if(u1 == 1)
  Constant : Constant
  Data Store Write : DataStoreWrite  DataStoreName=feedback_flag_18dim_RIEKF  IndexOptions=Index vector (dialog)  Indices=1  OutputSizes=1
  wires:
  Constant/1 -> Data Store Write/1

== system VB_RIFKF_GNSS_INS25/ISUS_RIEKF3/INS propogation3/Init_PVQ/Horizontal_attitude/Deal with zero ==
  In1 : Inport
  Add5 : Sum
  Constant1 : Constant  Value=1e-6  OutDataTypeStr=single
  Out1 : Outport
  wires:
  Add5/1 -> Out1/1
  In1/1 -> Add5/1
  Constant1/1 -> Add5/2

== system VB_RIFKF_GNSS_INS25/ISUS_RIEKF3/INS propogation3/gyro bias compensation/error compensation/If Action Subsystem1 ==
  Action Port : ActionPort  ActionPortLabel=if(u1 == 1)
  Constant : Constant
  Data Store Write : DataStoreWrite  DataStoreName=feedback_flag_18dim_RIEKF  IndexOptions=Index vector (dialog)  Indices=1  OutputSizes=1
  wires:
  Constant/1 -> Data Store Write/1

== matlab function VB_RIFKF_GNSS_INS25/ISUS_RIEKF2/Error State Kalman Filter M1/MATLAB Function ==
  data: u input; dp output size=3; dv output size=3; dtheta output size=3; da output size=3; dg output size=3
function [dp,dv,dtheta,da,dg] = fcn(u)
    dtheta = u(1:3);
    dv = u(4:6);
    dp = u(7:9);
    dg = u(10:12);
    da = u(13:15);

end

== matlab function VB_RIFKF_GNSS_INS25/ISUS_RIEKF1/Error State Kalman Filter M1/MATLAB Function ==
  data: u input; dp output size=3; dv output size=3; dtheta output size=3; da output size=3; dg output size=3
function [dp,dv,dtheta,da,dg] = fcn(u)
    dtheta = u(1:3);
    dv = u(4:6);
    dp = u(7:9);
    dg = u(10:12);
    da = u(13:15);

end

== matlab function VB_RIFKF_GNSS_INS25/ISUS_RIEKF1/Error State Kalman Filter M1/MATLAB Function1 ==
  data: u input; y output; time input
function y = fcn(u,time)
abs = 0;
if time > 60 && time < 61
    abs = 1000;
end
y = u + [abs;0;0];

== matlab function VB_RIFKF_GNSS_INS25/ISUS_RIEKF1/Error State Kalman Filter M1/MATLAB Function2 ==
  data: t input; u input; y output
function y = fcn(t,u)
if t<160
    s=1; 
    y = u;
else 
    s=10; 
    y = u + ([0.1;0.1;0.1].*htwn(0.1,s,3));
end

== matlab function VB_RIFKF_GNSS_INS25/No.1_Sensor_Data_Process/Magn_Data_Process/MATLAB Function1 ==
  data: u input; y output
function y = Normalization(u)
   dim = 3;
   y = zeros(dim,1);
y = double(u/sqrt(u(1)^2 + u(2)^2 + u(3)^2));

== matlab function VB_RIFKF_GNSS_INS25/read FC1_y/Subsystem2/MATLAB Function ==
  data: u input; y output; u_1 input
function y = fcn(u,u_1)
if abs(u) > 100
    y = u_1;
end
y = u;

== matlab function VB_RIFKF_GNSS_INS25/ISUS_RIEKF1/Error State Kalman Filter M1/Simulink Function - GPS Measurements/MATLAB Function ==
  data: vn input; H output; pn input
function H = fcn(vn, pn)
    state_dim = 15;
    H = zeros(6,state_dim);
    H(1:3,1:3) = skewMat(vn);
    H(4:6,1:3) = skewMat(pn);
    H(1:6,4:9) = eye(6);
    %H = -H;
end

== matlab function VB_RIFKF_GNSS_INS25/ISUS_RIEKF3/INS propogation2/att update/MATLAB Function2 ==
  data: delta input; Rbn_correct output single size=[3,3]; Rbn input
function Rbn_correct = fcn(delta, Rbn)
    Rbn_correct = zeros(3,3);
     Rbn_correct = exp_so3(delta)* Rbn;
    %Rbn_correct =( eye(3) + skewMat(delta))* Rbn;
end

== matlab function VB_RIFKF_GNSS_INS25/No.1_Sensor_Data_Process/Subsystem/TD_baro/MATLAB Function2 ==
  data: T input single; u1 output; u0 input; u1 input single; u2 input single; h input single; r input single; u2 output
function [u1,u2]=diff_TD_2(T,u0,u1,u2,h,r)
    %init
    %T是信号周期，u0原始信号输入，u1跟踪原始信号，u2原始信号差分值，
    %h滤波因子（h=T时接近一阶差分）越大滤波好延迟大；r速度因子，越大跟踪的越快但是噪声放大；

	x1=0; x2=0;
	delta=0;
	delta0=0;
	y=0;
	fabs_y=0;
	a0=0;
	a=0;
    fst=0;
    
	x1 = u1;
	x2 = u2;
	delta = r*h;
	delta0 = delta*h;
	y = x1 - u0 + h*x2;
	fabs_y = abs(y);   
	a0 = sqrt(delta*delta + 8 * r*fabs_y);
    
	if (fabs_y <= delta0)
		a = x2 + y / h;
    else
        a = x2 + 0.5*(a0 - delta)*sign(y);
    end
    
	if (abs(a) <= delta)
		fst = -r*a / delta;
    else
		fst = -r*sign(a);
    end
	u1 = single(x1 + T*x2); %计算跟踪信号
	u2 = single(x2 + T*fst); % 计算微分信号

== matlab function VB_RIFKF_GNSS_INS25/ISUS_RIEKF1/Error State Kalman Filter M1/Simulink Function - GPS Measurements/MATLAB Function1 ==
  data: Rbn input; vn input; X_inv output; pn input
function X_inv = invX(Rbn, vn, pn)
    X_inv = zeros(5,5);
    Rnb = Rbn';
    X_inv(1:3,1:3) = Rnb;
    X_inv(1:3,4) = -Rnb * vn;
    X_inv(1:3,5) = -Rnb * pn;
    X_inv(4:5,4:5) = eye(2);
end

== matlab function VB_RIFKF_GNSS_INS25/ISUS_RIEKF1/Error State Kalman Filter M1/Simulink Function - GPS Measurements1/MATLAB Function ==
  data: vn input; H_baro output; pn input
function H_baro = fcn(vn, pn)
    state_dim = 24;
    H = zeros(6,state_dim);
    H(1:3,1:3) = skewMat(vn);
    H(4:6,1:3) = skewMat(pn);
    H(1:6,4:9) = eye(6);
    
    A = [0 0 0 0 0 1];
    H_baro = A * H;
end

== matlab function VB_RIFKF_GNSS_INS25/ISUS_RIEKF1/Error State Kalman Filter M1/Simulink Function - GPS Measurements2/MATLAB Function ==
  data: Rbn input; Magn input; H output; dtheta input
function H = fcn(Rbn, Magn, dtheta)
    state_dim = 24;
    H = zeros(3,state_dim);
    H(1:3,1:3) =  Rbn * skewMat(Magn);
    H(1:3,16:18) =  Rbn * skewMat(dtheta);
end

== matlab function VB_RIFKF_GNSS_INS25/ISUS_RIEKF1/Error State Kalman Filter M1/Simulink Function - GPS Measurements3/MATLAB Function ==
  data: Rbn input; Rab input; H output; vn input; v_wind input
function H = fcn(Rbn,Rab, vn,v_wind)
    state_dim = 24;
    A = Rab' * Rbn';
    H = zeros(3,state_dim);
   % H(1:3,1:3) =  - skewMat(vn - v_wind);
   % H(1:3,4:6) =  eye(3);
    H(1:3,19:21) =  - skewMat(vn - v_wind);
    H(1:3,22:24) =  - eye(3);
    H = double(A * H);
end

== matlab function VB_RIFKF_GNSS_INS25/ISUS_RIEKF1/Error State Kalman Filter M1/Simulink Function - State Transition/Cal Phi/MATLAB Function1 ==
  data: vn input; Phi output; pn input; Rbn input; dt input
function Phi = fcn(vn,pn, Rbn,dt)
    state_dim = 15;
    %{
    F.block(0, 0, 3, 3) = exp_so3(-w_hat * dt);
        F.block(0, 9, 3, 3).noalias() = -exp_so3(-w_hat * dt) * Jr_so3(-w_hat * dt) * dt;
        F.block(9, 9, 3, 3).setIdentity();
        F.block(6, 0, 3, 3).noalias() = -R_Gtoi.transpose() * skew_x(a_hat * dt);
        F.block(6, 6, 3, 3).setIdentity();
        F.block(6, 12, 3, 3) = -R_Gtoi.transpose() * dt;
        F.block(12, 12, 3, 3).setIdentity();
        F.block(3, 0, 3, 3).noalias() = -0.5 * R_Gtoi.transpose() * skew_x(a_hat * dt * dt);
        F.block(3, 6, 3, 3) = Eigen::Matrix3d::Identity() * dt;
        F.block(3, 12, 3, 3) = -0.5 * R_Gtoi.transpose() * dt * dt;
        F.block(3, 3, 3, 3).setIdentity();
        Eigen::Matrix<double, 15, 12> G = Eigen::Matrix<double, 15, 12>::Zero();
    %}
    %
    %
    %F = [0_33         0_33  0_33   -Rbn          0_33]
    %    [skew(gn)     0_33  0_33  -skew(vn)Rbn   -Rbn]
    %    [0.5*skew(gn) I_33  0_33  -skew(pn)Rbn   -Rbn]
    %    [         0_69                  I66          ]
    %
    %0611 yxy
        %F = [0_33         0_33  0_33   -Rbn          0_33]
    %    [skew(gn)     0_33  0_33  -skew(vn)Rbn   Rbn]
    %    [0.5*skew(gn) I_33  0_33  -skew(pn)Rbn   Rbn]
    %    [         0_69                  I66          ]
    Phi = zeros(state_dim,state_dim);
    g0 = 9.79;
    gn = [0;0;-g0];
    tao_wind = 50;
    F  = zeros(state_dim,state_dim);
    F(1:3,10:12) = -Rbn;
    F(4:6,1:3)   = skewMat(gn);
    F(4:6,10:12) = -skewMat(vn)*Rbn;
    F(4:6,13:15) = -Rbn*(-1);
    F(7:9,4:6)   = eye(3);
    F(7:9,1:3)   = 0.5*skewMat(gn)*dt;
    F(7:9,10:12) = -skewMat(pn)*Rbn;
    F(7:9,13:15) = -Rbn*(-1);
    %F(10:15,10:15) = eye(6);
    % F(22:24,22:24) = -1/tao_wind;
    Phi = eye(state_dim) + F * dt;

end

== matlab function VB_RIFKF_GNSS_INS25/ISUS_RIEKF1/Error State Kalman Filter M1/Simulink Function - State Transition/MATLAB Function ==
  data: Rbn input; G output; vn input; pn input; dt input
function G = fcn(Rbn, vn,pn, dt)
    % G.block(0, 0, 3, 3) = -exp_so3(-w_hat * dt) * Jr_so3(-w_hat * dt) * dt;
    %    G.block(6, 3, 3, 3) = -R_Gtoi.transpose() * dt;
    %    G.block(3, 3, 3, 3) = -0.5 * R_Gtoi.transpose() * dt * dt;
    %    G.block(9, 6, 3, 3).setIdentity();
    %    G.block(12, 9, 3, 3).setIdentity();
    state_dim = 15;
    cov_dim = 12;
    G = zeros(state_dim,cov_dim);
    % G(1:3,1:3) = -  Rbn * dt;
    % G(4:6,1:3) = -skewMat(vn)*Rbn* dt;
    % G(4:6,4:6) =  - Rbn;
    % G(7:9,1:3) = -skewMat(pn)*Rbn * dt;
    % G(7:9,4:6) =  - Rbn;
    % G(10:12,7:9) = eye(3)*dt;
    % G(13:15,10:12) = eye(3)*dt;
    G(1:3,1:3) =  - Rbn * dt;
    G(4:6,1:3) = -skewMat(vn)*Rbn * dt*(-1);
    G(4:6,4:6) =  - Rbn * dt;
    G(7:9,1:3) = -skewMat(pn)*Rbn * dt*(-1);
    G(7:9,4:6) =  - Rbn * dt;
    G(10:12,7:9) = eye(3)* dt;
    G(13:15,10:12) = eye(3);
    % G(16:18,13:15) = eye(3);
    % G(19:21,16:18) = eye(3)* dt;
    % G(22:24,19:21) = eye(3)* dt;
    %G = G*double(dt);
end

== matlab function VB_RIFKF_GNSS_INS25/ISUS_RIEKF1/Error State Kalman Filter M1/Simulink Function - State Transition1/Cal Phi/MATLAB Function1 ==
  data: vn input; Phi output; pn input; Rbn input; dt input
function Phi = fcn(vn,pn, Rbn,dt)
    state_dim = 15;
    %{
    F.block(0, 0, 3, 3) = exp_so3(-w_hat * dt);
        F.block(0, 9, 3, 3).noalias() = -exp_so3(-w_hat * dt) * Jr_so3(-w_hat * dt) * dt;
        F.block(9, 9, 3, 3).setIdentity();
        F.block(6, 0, 3, 3).noalias() = -R_Gtoi.transpose() * skew_x(a_hat * dt);
        F.block(6, 6, 3, 3).setIdentity();
        F.block(6, 12, 3, 3) = -R_Gtoi.transpose() * dt;
        F.block(12, 12, 3, 3).setIdentity();
        F.block(3, 0, 3, 3).noalias() = -0.5 * R_Gtoi.transpose() * skew_x(a_hat * dt * dt);
        F.block(3, 6, 3, 3) = Eigen::Matrix3d::Identity() * dt;
        F.block(3, 12, 3, 3) = -0.5 * R_Gtoi.transpose() * dt * dt;
        F.block(3, 3, 3, 3).setIdentity();
        Eigen::Matrix<double, 15, 12> G = Eigen::Matrix<double, 15, 12>::Zero();
    %}
    %
    %
    %F = [0_33         0_33  0_33   -Rbn          0_33]
    %    [skew(gn)     0_33  0_33  -skew(vn)Rbn   -Rbn]
    %    [0.5*skew(gn) I_33  0_33  -skew(pn)Rbn   -Rbn]
    %    [         0_69                  I66          ]
    %
    %0611 yxy
        %F = [0_33         0_33  0_33   -Rbn          0_33]
    %    [skew(gn)     0_33  0_33  -skew(vn)Rbn   Rbn]
    %    [0.5*skew(gn) I_33  0_33  -skew(pn)Rbn   Rbn]
    %    [         0_69                  I66          ]
    Phi = zeros(state_dim,state_dim);
    g0 = 9.79;
    gn = [0;0;-g0];
    tao_wind = 50;
    F  = zeros(state_dim,state_dim);
    F(1:3,10:12) = -Rbn;
    F(4:6,1:3)   = skewMat(gn);
    F(4:6,10:12) = -skewMat(vn)*Rbn;
    F(4:6,13:15) = -Rbn*(-1);
    F(7:9,4:6)   = eye(3);
    F(7:9,1:3)   = 0.5*skewMat(gn)*dt;
    F(7:9,10:12) = -skewMat(pn)*Rbn;
    F(7:9,13:15) = -Rbn*(-1);
    %F(10:15,10:15) = eye(6);
    % F(22:24,22:24) = -1/tao_wind;
    Phi = double(eye(state_dim) + F * dt);

end

== matlab function VB_RIFKF_GNSS_INS25/ISUS_RIEKF3/INS propogation2/vel//pos update/pos update/MATLAB Function ==
  data: dtheta input; pos_correct output single; KFState_dp input; pos input
function pos_correct = fcn(dtheta, KFState_dp, pos)
    
     pos_correct =  KFState_dp + exp_so3(dtheta)*pos;
    %pos_correct = pos + KFState_dp - skewMat(pos)*dtheta;
    
end

== matlab function VB_RIFKF_GNSS_INS25/ISUS_RIEKF1/Error State Kalman Filter M1/Simulink Function - State Transition1/MATLAB Function ==
  data: Rbn input; G output; vn input; pn input; dt input
function G = fcn(Rbn, vn,pn, dt)
    % G.block(0, 0, 3, 3) = -exp_so3(-w_hat * dt) * Jr_so3(-w_hat * dt) * dt;
    %    G.block(6, 3, 3, 3) = -R_Gtoi.transpose() * dt;
    %    G.block(3, 3, 3, 3) = -0.5 * R_Gtoi.transpose() * dt * dt;
    %    G.block(9, 6, 3, 3).setIdentity();
    %    G.block(12, 9, 3, 3).setIdentity();
    state_dim = 15;
    cov_dim = 12;
    G = zeros(state_dim,cov_dim);
    % G(1:3,1:3) = -  Rbn * dt;
    % G(4:6,1:3) = -skewMat(vn)*Rbn* dt;
    % G(4:6,4:6) =  - Rbn;
    % G(7:9,1:3) = -skewMat(pn)*Rbn * dt;
    % G(7:9,4:6) =  - Rbn;
    % G(10:12,7:9) = eye(3)*dt;
    % G(13:15,10:12) = eye(3)*dt;
    G(1:3,1:3) =  - Rbn * dt;
    G(4:6,1:3) = -skewMat(vn)*Rbn * dt*(-1);
    G(4:6,4:6) =  - Rbn * dt;
    G(7:9,1:3) = -skewMat(pn)*Rbn * dt*(-1);
    G(7:9,4:6) =  - Rbn * dt;
    G(10:12,7:9) = eye(3)* dt;
    G(13:15,10:12) = eye(3);
    % G(16:18,13:15) = eye(3);
    % G(19:21,16:18) = eye(3)* dt;
    % G(22:24,19:21) = eye(3)* dt;
    %G = G*double(dt);
end
